simulink model "trim_simulation"  (R2024a)
settings: Solver=FixedStepAuto  StartTime=0.0  StopTime=10.0  RelTol=1e-3
settings Model: Creator=PC  LastModifiedBy=PC

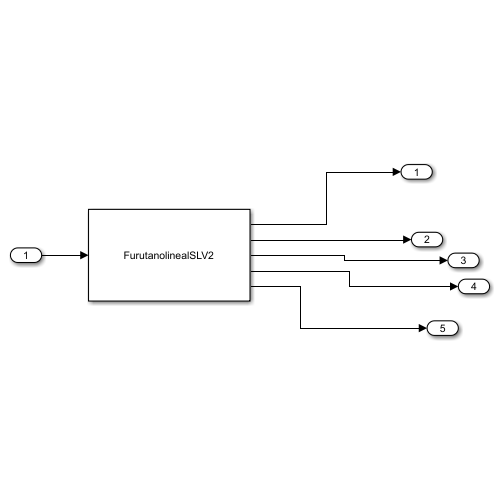
[thumbnail: Simulink's stored preview of the top-level diagram]
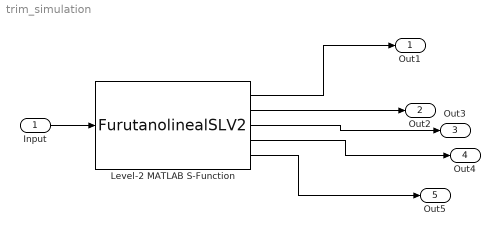
== system trim_simulation ==
  Input : Inport
  Level-2 MATLAB S-Function : M-S-Function  FunctionName=FurutanolinealSLV2
  Out1 : Outport
  Out2 : Outport  Port=2
  Out3 : Outport  Port=3
  Out4 : Outport  Port=4
  Out5 : Outport  Port=5
  wires:
  Input/1 -> Level-2 MATLAB S-Function/1
  Level-2 MATLAB S-Function/1 -> Out1/1
  Level-2 MATLAB S-Function/3 -> Out3/1
  Level-2 MATLAB S-Function/2 -> Out2/1
  Level-2 MATLAB S-Function/4 -> Out4/1
  Level-2 MATLAB S-Function/5 -> Out5/1
